simulink model "Junctions5_tmp"  (Simulink 8.3)
settings: Solver=ode45  StartTime=0.0  StopTime=10.0  RelTol=1e-3
settings Model: Creator=scaife  LastModifiedBy=bourbouh  CovSFcnEnable=on  ExtModeAutoUpdateStatusClock=off
settings DataIOCC: SignalLoggingName=sigsOut
settings DebuggingCC: SaveWithParameterizedLinksMsg=none  SignalResolutionControl=TryResolveAllWithWarning  SolverPrmCheckMsg=none  MultiTaskDSMMsg=warning  MultiTaskCondExecSysMsg=none  FrameProcessingCompatibilityMsg=error  StateNameClashWarn=none  StrictBusMsg=None
settings HardwareCC: TargetUnknown=on
settings SFSimCC: SimParseCustomCode=off
settings GRTTargetCC: GeneratePreprocessorConditionals=Use local settings

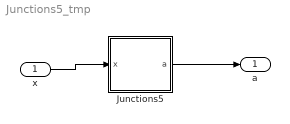
== system Junctions5_tmp ==
  x : Inport
  Junctions5 : Stateflow chart  TreatAsAtomicUnit=on
      settings: PermitHierarchicalResolution=ParametersOnly
  a : Outport
  wires:
  Junctions5/1(a) -> a/1
  x/1 -> Junctions5/1(x)

== stateflow chart Junctions5 ==
  state A/
    ex: a+=10000
  state B/
    ex: a=0
  (default) -> A
  A -> (junction 7) [order 2] : [x%%3==0]{a+=1}
  A -> (junction 7) [order 1] : [x%%3==1]{a+=10}
  (junction 7) -> (junction 8) : [x>=2]{a+=100}
  (junction 8) -> B : [x>=4]{a+=1000}
  data: x input int32; a output double
